simulink model "Project3_Part2C"  (R2020b)
settings: Solver=VariableStepAuto  StartTime=0.0  StopTime=10.0  RelTol=1e-3
settings Model: Creator=matth  LastModifiedBy=matth

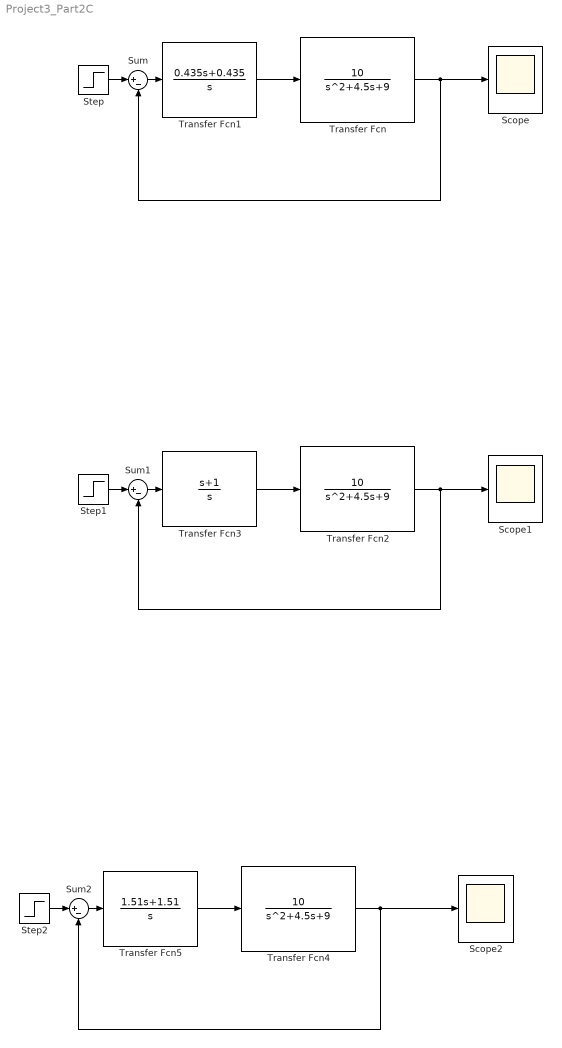
== system Project3_Part2C ==
  Scope : Scope
  Scope1 : Scope
  Scope2 : Scope
  Step : Step  SampleTime=0
  Step1 : Step  SampleTime=0
  Step2 : Step  SampleTime=0
  Sum : Sum  Inputs=|+-
  Sum1 : Sum  Inputs=|+-
  Sum2 : Sum  Inputs=|+-
  Transfer Fcn : TransferFcn  Numerator=[10]  Denominator=[1 4.5 9]
  Transfer Fcn1 : TransferFcn  Numerator=[0.435 0.435]  Denominator=[1 0]
  Transfer Fcn2 : TransferFcn  Numerator=[10]  Denominator=[1 4.5 9]
  Transfer Fcn3 : TransferFcn  Numerator=[1 1]  Denominator=[1 0]
  Transfer Fcn4 : TransferFcn  Numerator=[10]  Denominator=[1 4.5 9]
  Transfer Fcn5 : TransferFcn  Numerator=[1.51 1.51]  Denominator=[1 0]
  wires:
  Transfer Fcn1/1 -> Transfer Fcn/1
  Transfer Fcn/1 -> Sum/2, Scope/1
  Step/1 -> Sum/1
  Sum/1 -> Transfer Fcn1/1
  Sum1/1 -> Transfer Fcn3/1
  Step1/1 -> Sum1/1
  Transfer Fcn3/1 -> Transfer Fcn2/1
  Transfer Fcn2/1 -> Sum1/2, Scope1/1
  Sum2/1 -> Transfer Fcn5/1
  Step2/1 -> Sum2/1
  Transfer Fcn5/1 -> Transfer Fcn4/1
  Transfer Fcn4/1 -> Sum2/2, Scope2/1
